simulink model "movement"  (R2023b)
settings: Solver=VariableStepAuto  StartTime=0.0  StopTime=10  MaxStep=0.1  MinStep=0.1  RelTol=1e-3
settings Model: Creator=Yasmine Adler  LastModifiedBy=Yasmine Adler

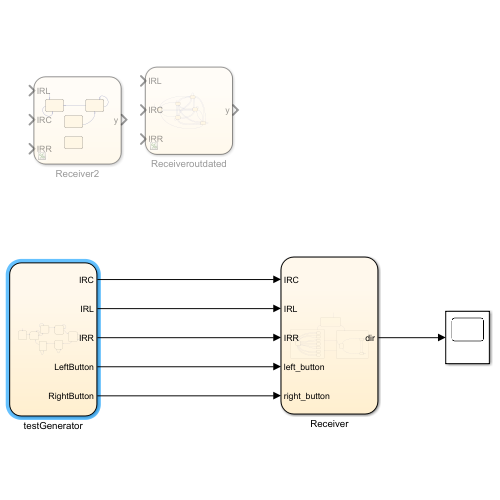
[thumbnail: Simulink's stored preview of the top-level diagram]
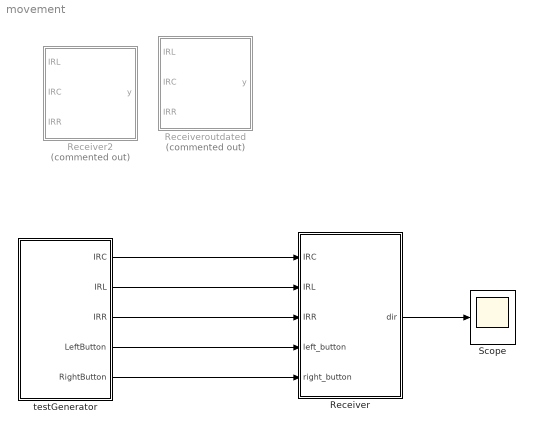
== system movement ==
  Receiver : Stateflow chart  TreatAsAtomicUnit=on
      settings: PortSchema="{\"entries\":[{\"content\":{\"sides\":[{\"content\":{\"connectorIds\":[\"In1\",\"In2\",\"In3\",\"In5\",\"In4\"]},\"type\":\"ConnectorPlacement.EquallySpacedRectSide\",\"uuid\":\"a7c67967-75fc-40e8-bf52-5a8169edc620\"},{\"content\":{\"connectorIds\":[\"Out1\"],\"side\":\"RIGHT\"},\"type\":\"ConnectorPlacement.EquallySpacedRectSide\",\"uuid\":\"0dd475c1-ea75-459f-a8c7-6ac5ab631be3\"},{\"content\":{\"side\":\"TOP\"},\"type\":\"ConnectorPlacement.EquallySpacedRectSide\",\"uuid\":\"2c10dc14-9c81-4037-bdaa-535c372efd5c\"}]},\"type\":\"ConnectorPlacement.EquallySpacedConnector\",\"uuid\":\"9b1f0b47-87eb-452b-974e-80cffe1332dc\"}],\"packageUris\":[\"http://schema.mathworks.com/mf0/Connector/R2020b\"],\"version\":\"1.0\"}"
  Receiver2 : Stateflow chart  Commented=on  TreatAsAtomicUnit=on
      settings: PortSchema="{\"entries\":[{\"content\":{\"sides\":[{\"content\":{\"connectorIds\":[\"In3\",\"In1\",\"In2\"]},\"type\":\"ConnectorPlacement.EquallySpacedRectSide\",\"uuid\":\"3e103536-5285-48a0-81ad-92eb0938af06\"},{\"content\":{\"connectorIds\":[\"Out1\"],\"side\":\"RIGHT\"},\"type\":\"ConnectorPlacement.EquallySpacedRectSide\",\"uuid\":\"b02ab8c7-8171-4867-a732-6e1e7f56a02e\"},{\"content\":{\"side\":\"TOP\"},\"type\":\"ConnectorPlacement.EquallySpacedRectSide\",\"uuid\":\"dbc7dc54-faab-4f8f-b4dd-69f62f45769e\"}]},\"type\":\"ConnectorPlacement.EquallySpacedConnector\",\"uuid\":\"ce3815ad-caf4-47cf-9a02-c941937ca115\"}],\"packageUris\":[\"http://schema.mathworks.com/mf0/Connector/R2020b\"],\"version\":\"1.0\"}"
  Receiveroutdated : Stateflow chart  Commented=on  TreatAsAtomicUnit=on
      settings: PortSchema="{\"entries\":[{\"content\":{\"sides\":[{\"content\":{\"connectorIds\":[\"In3\",\"In1\",\"In2\"]},\"type\":\"ConnectorPlacement.EquallySpacedRectSide\",\"uuid\":\"3e103536-5285-48a0-81ad-92eb0938af06\"},{\"content\":{\"connectorIds\":[\"Out1\"],\"side\":\"RIGHT\"},\"type\":\"ConnectorPlacement.EquallySpacedRectSide\",\"uuid\":\"b02ab8c7-8171-4867-a732-6e1e7f56a02e\"},{\"content\":{\"side\":\"TOP\"},\"type\":\"ConnectorPlacement.EquallySpacedRectSide\",\"uuid\":\"dbc7dc54-faab-4f8f-b4dd-69f62f45769e\"}]},\"type\":\"ConnectorPlacement.EquallySpacedConnector\",\"uuid\":\"ce3815ad-caf4-47cf-9a02-c941937ca115\"}],\"packageUris\":[\"http://schema.mathworks.com/mf0/Connector/R2020b\"],\"version\":\"1.0\"}"
  Scope : Scope
  testGenerator : Stateflow chart  TreatAsAtomicUnit=on
      settings: PortSchema="{\"entries\":[{\"content\":{\"sides\":[{\"content\":{},\"type\":\"ConnectorPlacement.EquallySpacedRectSide\",\"uuid\":\"6471699b-62f9-4f91-aa69-9d89f0e09012\"},{\"content\":{\"connectorIds\":[\"Out1\",\"Out3\",\"Out2\",\"Out5\",\"Out4\"],\"side\":\"RIGHT\"},\"type\":\"ConnectorPlacement.EquallySpacedRectSide\",\"uuid\":\"9e325bec-2460-4b35-8ca1-34a3b99ec345\"},{\"content\":{\"side\":\"TOP\"},\"type\":\"ConnectorPlacement.EquallySpacedRectSide\",\"uuid\":\"be98c419-042e-4242-8004-e979daadf4de\"}]},\"type\":\"ConnectorPlacement.EquallySpacedConnector\",\"uuid\":\"27bb65a1-fab6-45c1-b4f4-0c2a68e16e1c\"}],\"packageUris\":[\"http://schema.mathworks.com/mf0/Connector/R2020b\"],\"version\":\"1.0\"}"
  wires:
  Receiver/1(dir) -> Scope/1
  testGenerator/1(IRC) -> Receiver/1(IRC)
  testGenerator/2(IRR) -> Receiver/3(IRR)
  testGenerator/3(IRL) -> Receiver/2(IRL)
  testGenerator/4(RightButton) -> Receiver/4(right_button)
  testGenerator/5(LeftButton) -> Receiver/5(left_button)

== stateflow chart movement/Receiveroutdated ==
  state Right
    y=-2;
  state Midright
    y=-1;
  state idle
    y="idle";
  state Mid
    y=0;
  state Midleft
    y=1;
  state Left
    y=2;
  Right -> Right [order 1] : [IRL>TH && IRR>TH && IRC>TH]{noSig = noSig + 1}
  Right -> Left [order 4]
  idle -> Right [order 3] : [IRL]
  Right -> Midright [order 2]
  Left -> Right [order 2]
  Midright -> Right [order 2]
  Right -> Midleft [order 5]
  Midleft -> Right [order 3]
  Right -> Mid [order 3]
  Mid -> Right [order 2]
  Midright -> Midright [order 1] : [IRL>TH && IRR>TH && IRC>TH]{noSig = noSig + 1}
  idle -> Midright [order 4]
  (default) -> idle
  Midleft -> Midright [order 4]
  Midright -> Midleft [order 3]
  Left -> Midright [order 3]
  Midright -> Left [order 5]
  Mid -> Midright [order 3]
  Midright -> Mid [order 4]
  Mid -> Mid [order 1] : [IRL>TH && IRR>TH && IRC>TH]{noSig = noSig + 1}
  idle -> Mid [order 2] : [IRC<(IRL-TH2)&&IRC<(IRR-TH2)]
  Mid -> Left [order 4]
  idle -> Mid [order 1] : [IRL>TH && IRR>TH && IRC>TH]{noSig = noSig + 1}
  idle -> Left [order 6]
  idle -> Midleft [order 5]
  Mid -> Midleft [order 5]
  Midleft -> Mid [order 5]
  Left -> Mid [order 4]
  Midleft -> Midleft [order 2] : [IRL>TH && IRR>TH && IRC>TH]{noSig = noSig + 1}
  Midleft -> Left [order 1]
  Left -> Midleft [order 5]
  Left -> Left [order 1] : [IRL>TH && IRR>TH && IRC>TH]{noSig = noSig + 1}
  data: y output; IRC input; TH constant double =100; IRR input; noSig local; TH2 constant double =10; IRL input double

== stateflow chart movement/Receiver2 ==
  state MoveLeft
  state MoveRight
  state MoveCenter
  state Start
    IRL = 800
    IRC =
  (default) -> MoveLeft
  MoveRight -> MoveRight [order 2] : [x<5]
  MoveRight -> MoveLeft [order 1] : [x>=5]{x=0}
  MoveLeft -> MoveLeft : [x<5]
  MoveCenter -> MoveRight
  data: y output; IRC input; TH constant double =100; IRR input; noSig local; TH2 constant double =10; IRL input double

== stateflow chart movement/testGenerator ==
  state Setup
    count=0
    IRC = pres
    IRL = barpres
    IRR = barpres
    LeftButton = 0
    RightButton = 0
  state centerData
    IRC = pres
    IRL = barpres
    IRR = barpres
    LeftButton = 0
    RightButton = 0
  state MidRightData
    IRC = parpres
    IRL = barpres
    IRR = pres
    LeftButton = 0
    RightButton = 0
  state RightData
    IRC = barpres
    IRL = notpres
    IRR = pres
    LeftButton = 0
    RightButton = 0
  state LoseDataNoTrans
    IRC = notpres
    IRL = notpres
    IRR = notpres
    LeftButton = 0
    RightButton = 0
  state SwitchDir
    IRC = notpres
    IRL = notpres
    IRR = notpres
    LeftButton = 0
    RightButton = 0
  state MidLeftData
    IRC = parpres
    IRL = pres
    IRR = barpres
    LeftButton = 0
    RightButton = 0
  state LeftData
    IRC = barpres
    IRL = pres
    IRR = notpres
    LeftButton = 0
    RightButton = 0
  state ButtonPress
    IRC = notpres
    IRL = notpres
    IRR = notpres
    LeftButton = 1
    RightButton = 0
  state SwitchMode
    IRC = notpres
    IRL = notpres
    IRR = notpres
    LeftButton = 0
    RightButton = 0
  (default) -> Setup
  MidRightData -> MidRightData [order 2] : [count<num]{count = count + 1}
  centerData -> centerData [order 1] : [count<num]{count = count + 1}
  RightData -> RightData [order 2] : [count<num]{count = count + 1}
  MidRightData -> RightData [order 1] : [count==num]{count=0}
  Setup -> centerData
  RightData -> LoseDataNoTrans [order 1] : [count==num]{count=0}
  SwitchDir -> centerData [order 1] : [count==num]{count=0}
  centerData -> MidRightData [order 2] : [count==num]{count=0}
  LoseDataNoTrans -> LoseDataNoTrans [order 2] : [count<num]{count = count + 1}
  SwitchDir -> SwitchDir [order 2] : [count<num]{count = count + 1}
  LoseDataNoTrans -> MidLeftData [order 1] : [count==num]{count=0}
  ButtonPress -> SwitchDir [order 1] : [count==1]{count=0}
  MidLeftData -> LeftData [order 1] : [count==num]{count=0}
  LeftData -> SwitchMode [order 2] : [count==num]{count=0}
  SwitchMode -> ButtonPress [order 2] : [count==switchMode]{count=0}
  ButtonPress -> ButtonPress [order 2] : [count<1]{count = count + 1}
  LeftData -> LeftData [order 1] : [count<num]{count = count + 1}
  MidLeftData -> MidLeftData [order 2] : [count<num]{count = count + 1}
  SwitchMode -> SwitchMode [order 1] : [count<switchMode]{count = count + 1}
  data: IRC output; IRR output; IRL output double; num local =4; count local; RightButton output; LeftButton output; pres local =3000; parpres local =3030; barpres local =3300; notpres local =4000; switchMode constant double =36

== stateflow chart movement/Receiver ==
  state InitializingMode
  state TrackingMode
    state Unknown
      dir=prev_state;
    state Stop
      dir=0;
    state RightTrack
      dir=-2;
    state MidrightTrack
      dir=-1;
    state comp
    state MidTrack
      dir=0;
    state MidleftTrack
      dir=1;
    state LeftTrack
      dir=2;
    state Error
    comp -> Unknown [order 2] : [IRL>AbsTh && IRC>AbsTh && IRR>AbsTh]{no_start_bit = no_start_bit + 1}
    Unknown -> comp : [no_start_bit<16]
    Stop -> comp : {prev_state=0}
    comp -> Stop [order 1] : [left_button || right_button]
    comp -> RightTrack [order 4] : [IRR<IRC && IRR < IRL ]{no_start_bit=0}
    RightTrack -> comp : {prev_state = -2}
    comp -> MidrightTrack [order 3] : [abs(IRC-IRR) < SmTh && IRR<IRC && IRR < IRL]{no_start_bit=0}
    MidrightTrack -> comp : {prev_state = -1}
    comp -> MidTrack [order 7] : [IRC<IRL && IRC < IRR]{no_start_bit=0}
    MidTrack -> comp : {prev_state = 0}
    (default) -> comp
    comp -> MidleftTrack [order 5] : [abs(IRC-IRL) < SmTh && IRL<IRC && IRL < IRR]{no_start_bit=0}
    MidleftTrack -> comp : {prev_state = 1}
    Error -> comp
    comp -> Error [order 8] : {no_start_bit=0}
    LeftTrack -> comp : {prev_state = 2}
    comp -> LeftTrack [order 6] : [IRL<IRC && IRL < IRR]{no_start_bit=0}
  state ScanningMode
    state RightScan
      dir=-3;
    state startScan
    state LeftScan
      dir=3;
    startScan -> RightScan [order 1] : [prev_state==-2 || prev_state==-1 ]
    RightScan -> RightScan [order 2]
    LeftScan -> RightScan [order 1] : [left_button]
    RightScan -> LeftScan [order 1] : [right_button]
    (default) -> startScan
    startScan -> LeftScan [order 2]
    LeftScan -> LeftScan [order 2]
  (default) -> InitializingMode
  InitializingMode -> TrackingMode [order 1] : [IRC<AbsTh || IRL < AbsTh || IRR < AbsTh]
  InitializingMode -> ScanningMode [order 2]
  TrackingMode -> ScanningMode : [IRL>AbsTh && IRC>AbsTh && IRR>AbsTh && no_start_bit>=16]
  ScanningMode -> TrackingMode : [IRL< AbsTh || IRR<AbsTh || IRC<AbsTh]{no_start_bit=0}
  data: dir output; IRC input; SmTh local =50; AbsTh local =3600; no_start_bit local; IRL input; IRR input; right_button input; left_button input; prev_state local
